simulink model "CANNetwork"  (R2019a)
settings: Solver=VariableStepAuto  StartTime=0.0  StopTime=10.0  FixedStep=0.003  RelTol=1e-3
libraries: truetime x9, cstblocks x2
settings Model: Creator=Alvaro UAO  LastModifiedBy=Alvaro UAO

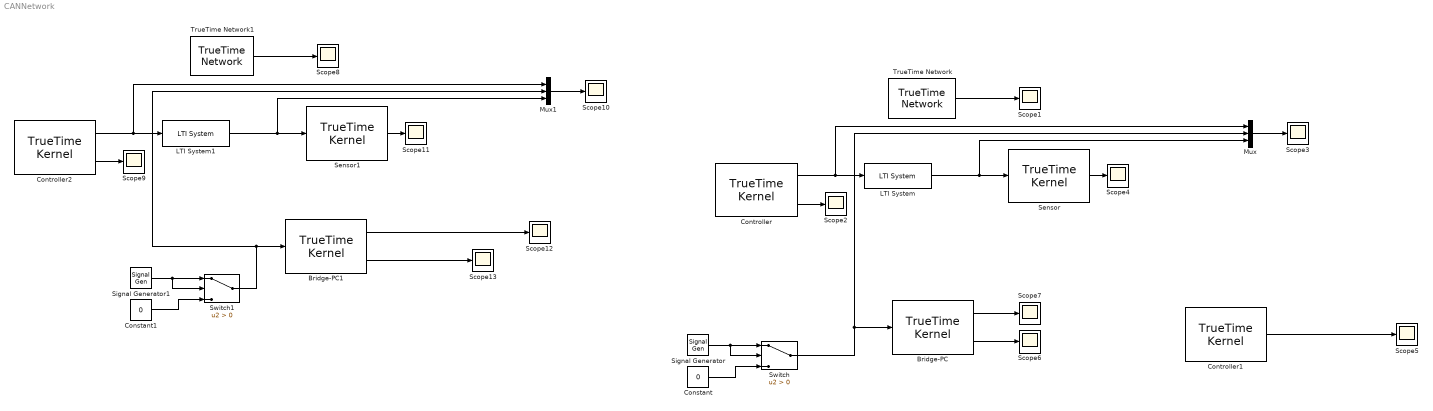
== system CANNetwork ==
  Bridge-PC : truetime/TrueTime Kernel  sfun=bridge_init  args=[]  ninputsoutputs=[1 1]  ntriggers=0  trigtype=falling  nwnodenbr=[1 3]  clockoffsetdrift=[0 0]  schedoutput=on  battery=off  poweroutput=off  label=1: 3
  Bridge-PC1 : truetime/TrueTime Kernel  sfun=bridge2_init  args=[]  ninputsoutputs=[1 1]  ntriggers=0  trigtype=falling  nwnodenbr=[2 3]  clockoffsetdrift=[0 0]  schedoutput=on  battery=off  poweroutput=off  label=2: 3
  Constant : Constant  Value=0
  Constant1 : Constant  Value=0
  Controller : truetime/TrueTime Kernel  sfun=controller_init  args=[]  ninputsoutputs=[0 1]  ntriggers=0  trigtype=falling  nwnodenbr=[1 2]  clockoffsetdrift=[0 0]  schedoutput=on  battery=off  poweroutput=off  label=1: 2
  Controller1 : truetime/TrueTime Kernel  sfun=disturbance_init  args=[]  ninputsoutputs=[0 0]  ntriggers=0  trigtype=falling  nwnodenbr=[1 4]  clockoffsetdrift=[0 0]  schedoutput=on  battery=off  poweroutput=off  label=1: 4
  Controller2 : truetime/TrueTime Kernel  sfun=controller_init  args=[]  ninputsoutputs=[0 1]  ntriggers=0  trigtype=falling  nwnodenbr=[2 2]  clockoffsetdrift=[0 0]  schedoutput=on  battery=off  poweroutput=off  label=2: 2
  LTI System : cstblocks/LTI System  sys=Quanzer  IC=[]
  LTI System1 : cstblocks/LTI System  sys=Quanzer  IC=[]
  Mux : Mux  Inputs=3
  Mux1 : Mux  Inputs=3
  Scope{1..13} (13 alike) : Scope
  Sensor : truetime/TrueTime Kernel  sfun=sensor_init  args=[]  ninputsoutputs=[1 0]  ntriggers=0  trigtype=falling  nwnodenbr=[1 1]  clockoffsetdrift=[0 0]  schedoutput=on  battery=off  poweroutput=off  label=1: 1
  Sensor1 : truetime/TrueTime Kernel  sfun=sensor_init  args=[]  ninputsoutputs=[1 0]  ntriggers=0  trigtype=falling  nwnodenbr=[2 1]  clockoffsetdrift=[0 0]  schedoutput=on  battery=off  poweroutput=off  label=2: 1
  Signal Generator : SignalGenerator  WaveForm=square  Amplitude=3  Frequency=0.2
  Signal Generator1 : SignalGenerator  WaveForm=square  Amplitude=3  Frequency=0.2
  Switch : Switch  Criteria=u2 > Threshold
  Switch1 : Switch  Criteria=u2 > Threshold
  TrueTime Network : truetime/TrueTime Network  nwtype=CSMA/CD (Ethernet)  nwnbr=1  nnodes=4  rate=250000  minsize=44  lossprob=0  seed=0  bandwidths=[0.5 0.5]  slotsize=512  schedule=[1 1 2]  memsize=80000  buftype=Common buffer  overflow=Retransmit  dynSchedule=0  miniSlotSize=0  NIT=0  QSortMode=FIFO  sync=0  irtSchedule=0  nrtLength=0  nodeGraph=0  scheduleoutput=on
  TrueTime Network1 : truetime/TrueTime Network  nwtype=CSMA/CD (Ethernet)  nwnbr=2  nnodes=4  rate=250000  minsize=44  lossprob=0  seed=0  bandwidths=[0.5 0.5]  slotsize=512  schedule=[1 1 2]  memsize=80000  buftype=Common buffer  overflow=Retransmit  dynSchedule=0  miniSlotSize=0  NIT=0  QSortMode=FIFO  sync=0  irtSchedule=0  nrtLength=0  nodeGraph=0  scheduleoutput=on
  wires:
  Controller/1 -> Mux/1, LTI System/1
  LTI System/1 -> Mux/3, Sensor/1
  TrueTime Network/1 -> Scope1/1
  Controller/2 -> Scope2/1
  Sensor/1 -> Scope4/1
  Bridge-PC/2 -> Scope6/1
  Bridge-PC/1 -> Scope7/1
  Mux/1 -> Scope3/1
  Signal Generator/1 -> Switch/2, Switch/1
  Constant/1 -> Switch/3
  Switch/1 -> Mux/2, Bridge-PC/1
  Controller1/1 -> Scope5/1
  Mux1/1 -> Scope10/1
  Sensor1/1 -> Scope11/1
  LTI System1/1 -> Mux1/3, Sensor1/1
  Bridge-PC1/2 -> Scope13/1
  Constant1/1 -> Switch1/3
  TrueTime Network1/1 -> Scope8/1
  Controller2/2 -> Scope9/1
  Controller2/1 -> Mux1/1, LTI System1/1
  Signal Generator1/1 -> Switch1/2, Switch1/1
  Switch1/1 -> Mux1/2, Bridge-PC1/1
  Bridge-PC1/1 -> Scope12/1
